simulink library "calcKalmanEstimate_ul"  (R2020a)
settings: Solver=VariableStepAuto  StartTime=0.0  StopTime=10.0  RelTol=1e-3
values from neighbouring files (symbols this model uses):
  hiLvlCtrl = block.DialogPrm(2).Data    [optimizeAltitude_Lvl2SFun.m]    (also in optimizeThrLenghtAndElevation_Lvl2sFun.m; optimizeTrajectory_Lvl2SFun.m)
  kfgp = block.DialogPrm(1).Data    [calcKalmanEstimate_Lvl2sFunc.m]    (also in calcKalmanEstimate_init.m = GP.KalmanFilteredGaussianProcess(hiLvlCtrl.spatialCovFn,    )
settings Model: Creator=Ayaz  LastModifiedBy=Ayaz

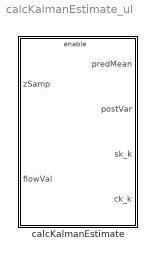
== system calcKalmanEstimate_ul ==
  calcKalmanEstimate : Subsystem  mask{hiLvlCtrl=hiLvlCtrl.kfgp}
      mask prompts: hiLvlCtrl "Hi-level controller object"
      mask init:
      | calcKalmanEstimate_init

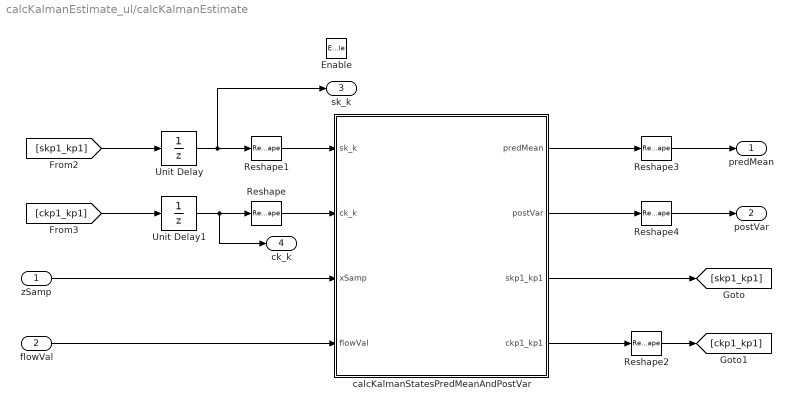
== system calcKalmanEstimate_ul/calcKalmanEstimate ==
  zSamp : Inport
  flowVal : Inport  Port=2
  Enable : EnablePort
  Reshape{,1,3..4} (4 alike) : Reshape  OutputDimensionality=Column vector (2-D)
  Reshape2 : Reshape  OutputDimensionality=Customize  OutputDimensions=length(kfgp.initVals.s0)*[1,1]
  Unit Delay : UnitDelay  InitialCondition=kfgp.initVals.s0  SampleTime=-1  HasFrameUpgradeWarning=on
  Unit Delay1 : UnitDelay  InitialCondition=kfgp.initVals.sig0Mat  SampleTime=-1  HasFrameUpgradeWarning=on
  calcKalmanStatesPredMeanAndPostVar : Subsystem
  predMean : Outport
  postVar : Outport  Port=2
  sk_k : Outport  Port=3
  ck_k : Outport  Port=4
  wires:
  calcKalmanStatesPredMeanAndPostVar/3(skp1_kp1) -> [skp1_kp1]
  calcKalmanStatesPredMeanAndPostVar/4(ckp1_kp1) -> Reshape2/1
  flowVal/1 -> calcKalmanStatesPredMeanAndPostVar/4(flowVal)
  calcKalmanStatesPredMeanAndPostVar/1(predMean) -> Reshape3/1
  calcKalmanStatesPredMeanAndPostVar/2(postVar) -> Reshape4/1
  Unit Delay/1 -> sk_k/1, Reshape1/1
  Unit Delay1/1 -> ck_k/1, Reshape/1
  [skp1_kp1] -> Unit Delay/1
  [ckp1_kp1] -> Unit Delay1/1
  Reshape/1 -> calcKalmanStatesPredMeanAndPostVar/2(ck_k)
  Reshape1/1 -> calcKalmanStatesPredMeanAndPostVar/1(sk_k)
  zSamp/1 -> calcKalmanStatesPredMeanAndPostVar/3(xSamp)
  Reshape2/1 -> [ckp1_kp1]
  Reshape3/1 -> predMean/1
  Reshape4/1 -> postVar/1

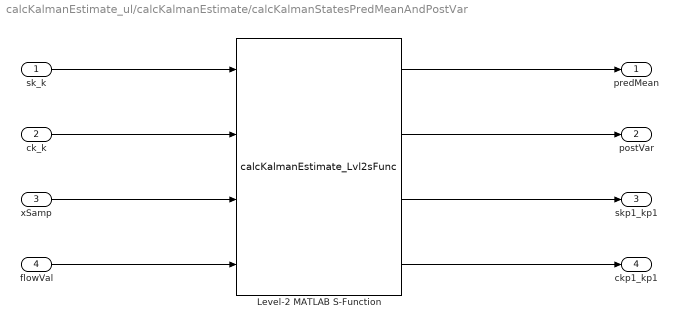
== system calcKalmanEstimate_ul/calcKalmanEstimate/calcKalmanStatesPredMeanAndPostVar ==
  sk_k : Inport
  ck_k : Inport  Port=2
  xSamp : Inport  Port=3
  flowVal : Inport  Port=4
  Level-2 MATLAB S-Function : M-S-Function  FunctionName=calcKalmanEstimate_Lvl2sFunc  Parameters=kfgp
  predMean : Outport
  postVar : Outport  Port=2
  skp1_kp1 : Outport  Port=3
  ckp1_kp1 : Outport  Port=4
  wires:
  xSamp/1 -> Level-2 MATLAB S-Function/3
  Level-2 MATLAB S-Function/2 -> postVar/1
  Level-2 MATLAB S-Function/1 -> predMean/1
  flowVal/1 -> Level-2 MATLAB S-Function/4
  Level-2 MATLAB S-Function/3 -> skp1_kp1/1
  Level-2 MATLAB S-Function/4 -> ckp1_kp1/1
  ck_k/1 -> Level-2 MATLAB S-Function/2
  sk_k/1 -> Level-2 MATLAB S-Function/1
